simulink model "CelpSimulink"  (Simulink 7.1)
settings: Solver=FixedStepDiscrete  StartTime=0.0  StopTime=inf  RelTol=1e-3
values from neighbouring files (symbols this model uses):
  codebook = [-2.05175223009 0.0511664262108 0.324261618767 1.39818550476 -0.777775598837 -0.917569683808 1.41237959687 2.97662916392 0.634067160969 0.306855989748 0.906306781051 0.102066164498 ... (20480 elements, 80x256)]    [codebook.mat]
undefined symbols (not defined in the file or in its folder): dfilt
libraries: dsparch4 x4, simulink x2, dspindex x2, dspsrcs4 x1, dsplp x1, dspbuff3 x1, dspsigops x1, dspstat3 x1, dspsnks4 x1
settings Model: Creator=Arthur  LastModifiedBy=Maquina
settings DebuggingCC: StrictBusMsg=ErrorLevel1

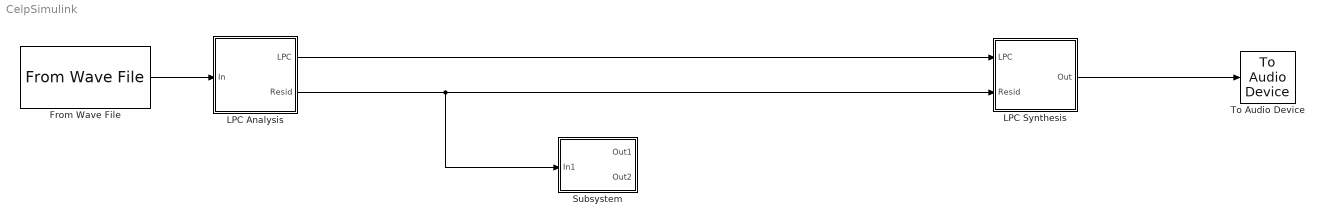
== system CelpSimulink ==
  From Wave File : dspsrcs4/From Wave File  FileName=audio.wav  SamplesPerFrame=80  MinBufSize=80  dType=single  bLoop=off  timesToPlay=1  restartMode=immediately after last sample  firstSampleOutput=off  lastSampleOutput=off
  LPC Analysis : Subsystem  Priority=1
  LPC Synthesis : Subsystem  Priority=3
  Subsystem : Subsystem  Priority=2
  To Audio Device : dspsnks4/To Audio Device  DialogController=dspDDGCreate  DialogControllerArgs=DataTag6  deviceName=Default  inheritSampleRate=off  sampleRate=8000  deviceDatatype=Determine from input data type  autoBufferSize=on  bufferSize=4096  queueDuration=1
  wires:
  LPC Analysis/1(LPC) -> LPC Synthesis/1(LPC)
  LPC Synthesis/1(Out) -> To Audio Device/1
  From Wave File/1 -> LPC Analysis/1(In)
  LPC Analysis/2(Resid) -> LPC Synthesis/2(Resid), Subsystem/1(In1)

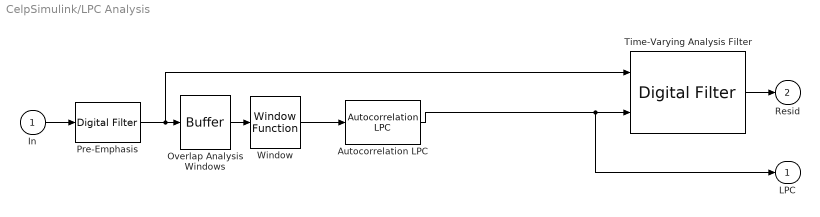
== system CelpSimulink/LPC Analysis ==
  In : Inport  OutDataType=sfix(16)  OutScaling=2^0
  Autocorrelation LPC : dsplp/Autocorrelation LPC  SystemSampleTime=-1  lpcCoeffOutFcn=A  lpcOutP=off  inherit_prediction_order=off  order=10
  Overlap Analysis Windows : dspbuff3/Buffer  N=160  V=80  ic=0
  Pre-Emphasis : dsparch4/Digital Filter  DialogController=dspdialog.DigitalFilter  DialogControllerArgs=DataTag0  TypePopup=FIR (all zeros)  IIRFiltStruct=Direct form II transposed  AllPoleFiltStruct=Direct form  FIRFiltStruct=Direct form  CoeffSource=Specify via dialog  NumCoeffs=[1 -.95] / 3.0  DenCoeffs=[1 0.1]  BiQuadCoeffs=[1 0.3 0.4 1 0.1 0.2]  LatticeCoeffs=[0.2 0.4]  denIgnore=on  FiltPerSampPopup=One filter per frame  IC=0  ICnum=0  ICden=0  roundingMode=Floor  overflowMode=off  ScaleValues=1  scaleValueFracLength=14  stageInFracLength=15  stageOutFracLength=15  FilterSource=Specify via dialog  dfiltObjectName=dfilt.dffir([1 2 1])
  Time-Varying Analysis Filter : dsparch4/Digital Filter  DialogController=dspdialog.DigitalFilter  DialogControllerArgs=DataTag1  TypePopup=FIR (all zeros)  IIRFiltStruct=Direct form II transposed  AllPoleFiltStruct=Direct form  FIRFiltStruct=Direct form  CoeffSource=Input port(s)  NumCoeffs=[1 -.95] / 3.0  DenCoeffs=[1 0.1]  BiQuadCoeffs=[1 0.3 0.4 1 0.1 0.2]  LatticeCoeffs=[0.2 0.4]  denIgnore=on  FiltPerSampPopup=One filter per frame  IC=0  ICnum=0  ICden=0  roundingMode=Floor  overflowMode=off  ScaleValues=1  scaleValueFracLength=14  stageInFracLength=15  stageOutFracLength=15  FilterSource=Input port(s)  dfiltObjectName=dfilt.dffir([1 2 1])
  Window : dspsigops/Window Function  DialogController=dspDDGCreate  DialogControllerArgs=DataTag2  winmode=Apply window to input  wintype=Hamming  sampmode=Continuous  samptime=1  N=64  Rs=50  beta=10  winsamp=Symmetric  UserWindow=hamming  OptParams=off  UserParams={1.0}  dataType=double  isSigned=on  wordLen=16  udDataType=sfix(16)  fracBitsMode=Best precision  numFracBits=15  roundingMode=Floor  overflowMode=off  numSidelobes=4  sidelobeLevel=-30
  LPC : Outport  OutDataType=sfix(16)  OutScaling=2^0
  Resid : Outport  Port=2  OutDataType=sfix(16)  OutScaling=2^0
  wires:
  Pre-Emphasis/1 -> Overlap Analysis Windows/1, Time-Varying Analysis Filter/1
  Overlap Analysis Windows/1 -> Window/1
  Autocorrelation LPC/1 -> LPC/1, Time-Varying Analysis Filter/2
  In/1 -> Pre-Emphasis/1
  Time-Varying Analysis Filter/1 -> Resid/1
  Window/1 -> Autocorrelation LPC/1

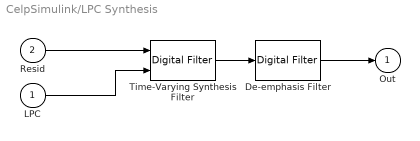
== system CelpSimulink/LPC Synthesis ==
  LPC : Inport  OutDataType=sfix(16)  OutScaling=2^0
  Resid : Inport  Port=2  OutDataType=sfix(16)  OutScaling=2^0
  De-emphasis Filter : dsparch4/Digital Filter  DialogController=dspdialog.DigitalFilter  DialogControllerArgs=DataTag3  TypePopup=IIR (all poles)  IIRFiltStruct=Direct form II transposed  AllPoleFiltStruct=Direct form  FIRFiltStruct=Direct form  CoeffSource=Specify via dialog  NumCoeffs=[1 -.95] / 3.0  DenCoeffs=[1 -.95]  BiQuadCoeffs=[1 0.3 0.4 1 0.1 0.2]  LatticeCoeffs=[0.2 0.4]  denIgnore=on  FiltPerSampPopup=One filter per frame  IC=0  ICnum=0  ICden=0  roundingMode=Floor  overflowMode=off  ScaleValues=1  scaleValueFracLength=14  stageInFracLength=15  stageOutFracLength=15  FilterSource=Specify via dialog  dfiltObjectName=dfilt.dffir([1 2 1])
  Time-Varying Synthesis Filter : dsparch4/Digital Filter  DialogController=dspdialog.DigitalFilter  DialogControllerArgs=DataTag4  TypePopup=IIR (all poles)  IIRFiltStruct=Direct form II transposed  AllPoleFiltStruct=Direct form  FIRFiltStruct=Direct form  CoeffSource=Input port(s)  NumCoeffs=[1 -.95] / 3.0  DenCoeffs=[1 0.1]  BiQuadCoeffs=[1 0.3 0.4 1 0.1 0.2]  LatticeCoeffs=[0.2 0.4]  denIgnore=off  FiltPerSampPopup=One filter per frame  IC=0  ICnum=0  ICden=0  roundingMode=Floor  overflowMode=off  ScaleValues=1  scaleValueFracLength=14  stageInFracLength=15  stageOutFracLength=15  FilterSource=Input port(s)  dfiltObjectName=dfilt.dffir([1 2 1])
  Out : Outport  OutDataType=sfix(16)  OutScaling=2^0
  wires:
  Time-Varying Synthesis Filter/1 -> De-emphasis Filter/1
  Resid/1 -> Time-Varying Synthesis Filter/1
  LPC/1 -> Time-Varying Synthesis Filter/2
  De-emphasis Filter/1 -> Out/1

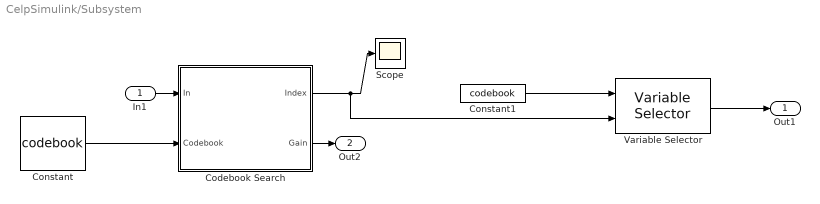
== system CelpSimulink/Subsystem ==
  In1 : Inport
  Codebook Search : Subsystem
  Constant : Constant  Value=codebook  OutDataTypeMode=single  OutDataType=fixdt(1, 16)  OutScaling=2^0  OutDataTypeStr=single
  Constant1 : Constant  Value=codebook  OutDataTypeMode=single  OutDataType=fixdt(1, 16)  OutScaling=2^0  OutDataTypeStr=single
  Scope : Scope
      settings: YMin=0  YMax=80
  Variable Selector : dspindex/Variable Selector  NumInputs=1  rowsOrCols=Columns  IdxMode=Variable  Elements=[1 3]  ZerOneIdxMode=One-based  errmode=Generate Error  FillMode=on  FillValues=0
  Out1 : Outport
  Out2 : Outport  Port=2
  wires:
  Constant/1 -> Codebook Search/2(Codebook)
  Codebook Search/1(Index) -> Scope/1, Variable Selector/2
  Constant1/1 -> Variable Selector/1
  In1/1 -> Codebook Search/1(In)
  Variable Selector/1 -> Out1/1
  Codebook Search/2(Gain) -> Out2/1

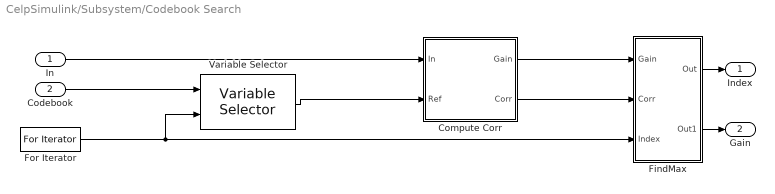
== system CelpSimulink/Subsystem/Codebook Search ==
  In : Inport
  Codebook : Inport  Port=2
  Compute Corr : Subsystem
  FindMax : Subsystem
  For Iterator : ForIterator  ResetStates=reset  IterationLimit=80
  Variable Selector : dspindex/Variable Selector  NumInputs=1  rowsOrCols=Columns  IdxMode=Variable  Elements=[1 3]  ZerOneIdxMode=One-based  errmode=Generate Error  FillMode=on  FillValues=0
  Index : Outport  OutDataType=fixdt(1, 16)  OutScaling=2^0
  Gain : Outport  Port=2  OutDataType=fixdt(1, 16)  OutScaling=2^0
  wires:
  Codebook/1 -> Variable Selector/1
  For Iterator/1 -> Variable Selector/2, FindMax/3(Index)
  FindMax/1(Out) -> Index/1
  In/1 -> Compute Corr/1(In)
  Variable Selector/1 -> Compute Corr/2(Ref)
  Compute Corr/1(Gain) -> FindMax/1(Gain)
  FindMax/2(Out1) -> Gain/1
  Compute Corr/2(Corr) -> FindMax/2(Corr)

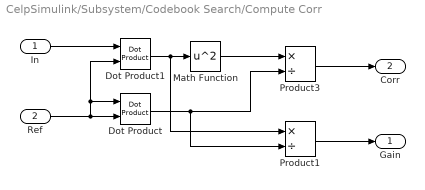
== system CelpSimulink/Subsystem/Codebook Search/Compute Corr ==
  In : Inport
  Ref : Inport  Port=2
  Dot Product : simulink/Math Operations/Dot Product  InputSameDT=on  OutDataType=sfix(16)  OutScaling=2^-10  DoSatur=off
  Dot Product1 : simulink/Math Operations/Dot Product  InputSameDT=on  OutDataType=sfix(16)  OutScaling=2^-10  DoSatur=off
  Math Function : Math  Operator=square  OutDataType=sfix(16)  OutScaling=2^0  SaturateOnIntegerOverflow=on
  Product1 : Product  Inputs=*/  OutDataType=sfix(16)  OutScaling=2^0  SaturateOnIntegerOverflow=on  OutDataTypeStr=Inherit: Same as first input
  Product3 : Product  Inputs=*/  OutDataType=sfix(16)  OutScaling=2^0  SaturateOnIntegerOverflow=on  OutDataTypeStr=Inherit: Same as first input
  Gain : Outport
  Corr : Outport  Port=2
  wires:
  Product1/1 -> Gain/1
  Ref/1 -> Dot Product/2, Dot Product/1, Dot Product1/2
  In/1 -> Dot Product1/1
  Dot Product1/1 -> Math Function/1, Product1/1
  Math Function/1 -> Product3/1
  Dot Product/1 -> Product3/2, Product1/2
  Product3/1 -> Corr/1

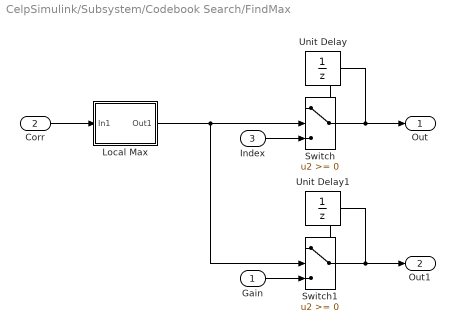
== system CelpSimulink/Subsystem/Codebook Search/FindMax ==
  Gain : Inport
  Corr : Inport  Port=2
  Index : Inport  Port=3
  "Local Max " : Subsystem
  Switch : Switch  OutDataType=fixdt(1, 16)  OutScaling=2^0
  Switch1 : Switch  OutDataType=fixdt(1, 16)  OutScaling=2^0
  Unit Delay : UnitDelay  SampleTime=-1
  Unit Delay1 : UnitDelay  SampleTime=-1
  Out : Outport
  Out1 : Outport  Port=2
  wires:
  Switch/1 -> Unit Delay/1, Out/1
  Unit Delay/1 -> Switch/1
  "Local Max "/1(Out1) -> Switch/2, Switch1/2
  Corr/1 -> "Local Max "/1(In1)
  Index/1 -> Switch/3
  Switch1/1 -> Unit Delay1/1, Out1/1
  Unit Delay1/1 -> Switch1/1
  Gain/1 -> Switch1/3

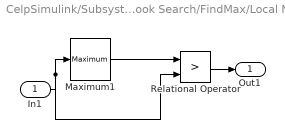
== system CelpSimulink/Subsystem/Codebook Search/FindMax/Local Max  ==
  In1 : Inport
  Maximum1 : dspstat3/Maximum  DialogController=dspfixptddg.MinMax  DialogControllerArgs=DataTag5  fcn=Running  reset=None  indexBase=One  operateOver=Each column  Dimension=1  colComp=on  operation=maximum  roundingMode=Floor  overflowMode=off
  Relational Operator : RelationalOperator  Operator=>  LogicOutDataTypeMode=boolean  LogicDataType=fixdt(0, 8)  OutDataTypeStr=boolean
  Out1 : Outport
  wires:
  In1/1 -> Maximum1/1, Relational Operator/2
  Maximum1/1 -> Relational Operator/1
  Relational Operator/1 -> Out1/1
